simulink model "IEEE13bus_1subsystem"  (R2022b)
settings: Solver=ode4  StartTime=0.0  StopTime=inf  FixedStep=Ts  MaxStep=1e-4  RelTol=1e-4
InitFcn:
  | a=1; % Loading Factor
  | Ts=50e-6;
  | % phase to sequence conversion of RXB matrices
  | c=1*exp(sqrt(-1)*(120*pi/180));
  | T=[1 1 1;1 c*c c;1 c c*c];
  | Tinv=1/3*[1 1 1;1 c c*c;1 c*c c];
  | 
  | % Simulation data for the IEEE 13 Node Test Feeder model
  | mi2km = 1.60934;%  miles to km conversion
  | ft2km = 0.0003048; % feet to km conversion
  | ms2F = 1*1e-6/(2*pi*60);% microsiemens to Farads conversion
  | 
  | 
  | %% Configuration 601
  | % Series Resitance and Reactance - ohm/mile
  | R_601 = [0.3465 0.1560 0.1580;0.1560 0.3375 0.1535;0.1580 0.1535 0.3414];
  | X_601 = [1.1079 0.5017 0.4236;0.5017 1.0478 0.3849;0.4236 0.3849 1.0348];
  | % charging susceptance - microsiemens/mile
  | B_601 = [6.2998 -1.9958 -1.2595;-1.9958 5.9597 -0.7417;-1.2595 -0.7417 5.6386];
  | 
  | R_601 = R_601/mi2km;
  | Rseq=Tinv*R_601*T;
  | R1_601=Rseq(2,2);R0_601=Rseq(1,1);
  | 
  | L_601 = (X_601/(2*pi*60))/mi2km;
  | Lseq=Tinv*L_601*T;
  | L1_601=Lseq(2,2);L0_601=Lseq(1,1);
  | 
  | C_601 =(B_601*ms2F)/mi2km;
  | Cseq=Tinv*C_601*T;
  | C1_601=Cseq(2,2);C0_601=Cseq(1,1);
  | 
  | %% Configuration 602 - series reactance - ohm/mile
  | R_602 = [0.7526 0.1580 0.1560;0.1580 0.7475 0.1535;0.1560 0.1535 0.7436];
  | X_602 = [1.1814 0.4236 0.5017;0.4236 1.1983 0.3849;0.5017 0.3849 1.2112];
  | % charging susceptance - microsiemens/mile
  | B_602 = [5.6990 -1.0817 -1.6905;-1.0817 5.1795 -0.6588;-1.6905 -0.6588 5.4246];
  | 
  | R_602 = R_602/mi2km;
  | Rseq=Tinv*R_602*T;
  | R1_602=Rseq(2,2);R0_602=Rseq(1,1);
  | 
  | L_602 = (X_602/(2*pi*60))/mi2km;
  | Lseq=Tinv*L_602*T;
  | L1_602=Lseq(2,2);L0_602=Lseq(1,1);
  | 
  | C_602 =(B_602*ms2F)/mi2km;
  | Cseq=Tinv*C_602*T;
  | C1_602=Cseq(2,2);C0_602=Cseq(1,1);
  | %% Configuration 603 - series reactance - ohm/mile
  | R_603 = [0 0 0;0 1.3294 0.2066;0 0.2066 1.3238];
  | X_603 = [0 0 0;0 1.3471 0.4591;0 0.4591 1.3569];
  | % charging susceptance - microsiemens/mile
  | B_603 = [0 0 0;0 4.7097 -0.8999;0 -0.8999 4.6658];
  | 
  | % convert for SPS
  | R_603 = R_603/mi2km;
  | Rseq=Tinv*R_603*T;
  | R1_603=Rseq(2,2);R0_603=Rseq(1,1);
  | 
  | ... (+71 lines)
undefined symbols (not defined in the file): find_system, I, Left, MOV_segment9, powergui, Right, type, V, X
libraries: spsSeriesRLCBranchLib x57, spsGroundLib x42, spsVoltageMeasurementLib x18, spsThreePhaseVIMeasurementLib x16, spsDCVoltageSourceLib x12, spsThreePhaseSeriesRLCLoadLib x7, ssn_lib x6, spsACCurrentSourceLib x6, spsOnDelayLib x6, spsThreePhasePISectionLineLib x5, spsSeriesRLCLoadLib x5, spsRMSLib x4
(part 4 of 4)

== system IEEE13bus_1subsystem/SM_13p/Regulator 1/Single Phase SVR_A2/Voltage Regulator Control/Tap Changer Control ==
  "Up " : Inport
  "Down " : Inport  Port=2
  Constant : Constant  Value=-1
  Constant1 : Constant
  Determine tap position : Subsystem
  Edge Detector : Subsystem  DialogController=POWERSYS.PowerSysDialog  mask(Edge Detector){model=Rising, ic=0}
      mask prompts: model "Edge:"; ic "Input at t = -eps:"
      mask help:
      | This block compares its present input to its previous input.
      |
      | If the input  is a logic signal (TRUE (1) or FALSE (0), the output is a one-step boolean signal TRUE  when  the specified edge (Rising, Falling or Either)  is detected.
      |
      | This block can also be used to detect the slope polarity of a continuous signal. For example, if the specified edge is  "Rising", the output is TRUE as long as the slope of the input signal is positive.
      |
      | The input value at time preceding t=0 is specified by the parameter "Input at t=-eps"
      mask init: same as IEEE13bus_1subsystem/SM_13p/Regulator 1/Single Phase SVR_A/Voltage Regulator Control/Tap Changer Control/Edge Detector
      mask Help: This block is part of a subset of blocks in the Extras library that does not have documentation associated with it, other than the block mask description.
      mask TypeOptions model: Rising | Falling | Either
      mask Display: plot(0,0,100,100, X1,Y1,X2,Y2,X3,Y3,X4,Y4);
  Logical Operator : Logic  Operator=OR  AllPortsSameDT=off
  Logical Operator1 : Logic  AllPortsSameDT=off
  Mechanical Delay : TransportDelay  DelayTime=MecDelay  InitialOutput=InitialPosition  BufferSize=5120
  Memory : Memory  InitialCondition=1  InheritSampleTime=on
  Relational Operator : RelationalOperator  Operator===  OutDataTypeStr=float('double')  InputSameDT=off
  Switch : Switch  Threshold=0.5  InputSameDT=off
  TapNo : Outport  VectorParamsAs1DForOutWhenUnconnected=off
  Ready : Outport  Port=2  VectorParamsAs1DForOutWhenUnconnected=off
  wires:
  Mechanical Delay/1 -> TapNo/1, Relational Operator/2
  Logical Operator1/1 -> Determine tap position/Trigger
  "Up "/1 -> Logical Operator/1
  "Down "/1 -> Logical Operator/2, Switch/2
  Constant/1 -> Switch/1
  Constant1/1 -> Switch/3
  Switch/1 -> Determine tap position/1(NewTap)
  Determine tap position/1(TapNo) -> Mechanical Delay/1, Relational Operator/1
  Relational Operator/1 -> Memory/1
  Memory/1 -> Logical Operator1/1, Ready/1
  Logical Operator/1 -> Edge Detector/1(In)
  Edge Detector/1(Out) -> Logical Operator1/2

== system IEEE13bus_1subsystem/SM_13p/Regulator 1/Single Phase SVR_A2/Voltage Regulator Control/Voltage regulator ==
  Vmes (pu) : Inport
  Ready : Inport  Port=2
  RegOn : Inport  Port=3
  Dead Zone : DeadZone  LowerValue=-DeadBand/2  UpperValue=+DeadBand/2
  Discrete Variable Time Delay : spsDiscreteVariableTimeDelayLib/Discrete Variable Time Delay  MaxDelay=3/60+Ts  InitialValue=1  Ts=Ts  DFT=on
      settings: LibrarySourceBlock=|
      | sps_lib/Control/Discrete Variable
      | Time Delay
  Logical Operator : Logic  AllPortsSameDT=off
  Logical Operator1 : Logic  AllPortsSameDT=off
  On Delay : spsOnDelayLib/On Delay  DelayType=On delay  delay=TimeDelay  ic=0  Ts=Ts
  On Delay1 : spsOnDelayLib/On Delay  DelayType=On delay  delay=TimeDelay  ic=0  Ts=Ts
  Relational Operator : RelationalOperator  Operator=>  InputSameDT=off
  Relational Operator1 : RelationalOperator  Operator=<  InputSameDT=off
  Sum : Sum  Inputs=|+-  SaturateOnIntegerOverflow=on
  Switch : Switch  Threshold=1.5  InputSameDT=off
  Vref : Constant  Value=Vref
  Vref1 : Constant  Value=0
  Vref2 : Constant  Value=0
  Vref3 : Constant  Value=0
  Vref4 : Constant  Value=3/60
  Up : Outport  VectorParamsAs1DForOutWhenUnconnected=off
  Down : Outport  Port=2  VectorParamsAs1DForOutWhenUnconnected=off
  wires:
  Vref2/1 -> Switch/3
  RegOn/1 -> Switch/2
  Switch/1 -> Dead Zone/1
  Sum/1 -> Switch/1
  Vref/1 -> Sum/1
  Vmes (pu)/1 -> Sum/2
  Dead Zone/1 -> Relational Operator1/1, Relational Operator/1
  Vref1/1 -> Relational Operator/2
  Relational Operator/1 -> Logical Operator/1
  Ready/1 -> Discrete Variable Time Delay/1
  Logical Operator/1 -> On Delay/1
  On Delay/1 -> Up/1
  Relational Operator1/1 -> Logical Operator1/2
  Logical Operator1/1 -> On Delay1/1
  On Delay1/1 -> Down/1
  Vref3/1 -> Relational Operator1/2
  Discrete Variable Time Delay/1 -> Logical Operator1/1, Logical Operator/2
  Vref4/1 -> Discrete Variable Time Delay/2

== system IEEE13bus_1subsystem/SM_13p/Regulator 1/Single Phase SVR_A/Transformer with Taps/SSN OLTC xfo v2/DC source_a ==
  I1A_V : spsDCVoltageSourceLib/DC Voltage Source  Amplitude=0  Measurements=None
  Conn1 : PMIOPort  Side=Left
  Conn2 : PMIOPort  Port=2  Side=Right
  connections:
  Conn2/RConn1 -- I1A_V/RConn1
  Conn1/RConn1 -- I1A_V/LConn1

== system IEEE13bus_1subsystem/SM_13p/Regulator 1/Single Phase SVR_A/Transformer with Taps/SSN OLTC xfo v2/DC source_b ==
  I1B_V : spsDCVoltageSourceLib/DC Voltage Source  Amplitude=0  Measurements=None
  Conn3 : PMIOPort  Side=Left
  Conn4 : PMIOPort  Port=2  Side=Right
  connections:
  Conn3/RConn1 -- I1B_V/LConn1
  Conn4/RConn1 -- I1B_V/RConn1

== system IEEE13bus_1subsystem/SM_13p/Regulator 1/Single Phase SVR_A/Transformer with Taps/SSN OLTC xfo v2/DC source_c ==
  I1C_V : spsDCVoltageSourceLib/DC Voltage Source  Amplitude=0  Measurements=None
  Conn1 : PMIOPort  Side=Left
  Conn2 : PMIOPort  Port=2  Side=Right
  connections:
  Conn1/RConn1 -- I1C_V/LConn1
  Conn2/RConn1 -- I1C_V/RConn1

== system IEEE13bus_1subsystem/SM_13p/Regulator 1/Single Phase SVR_A/Transformer with Taps/SSN OLTC xfo v2/DC source_d ==
  I1D_V : spsDCVoltageSourceLib/DC Voltage Source  Amplitude=0  Measurements=None
  Conn3 : PMIOPort  Side=Left
  Conn4 : PMIOPort  Port=2  Side=Right
  connections:
  Conn4/RConn1 -- I1D_V/RConn1
  Conn3/RConn1 -- I1D_V/LConn1

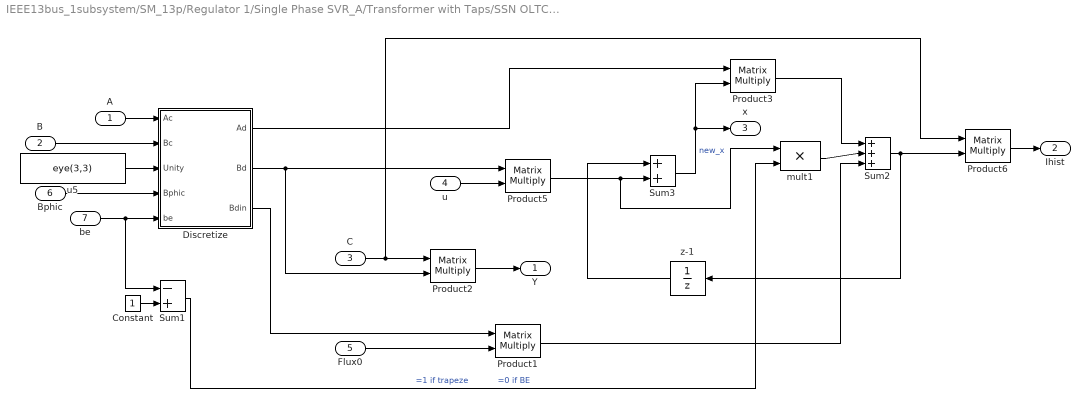
== system IEEE13bus_1subsystem/SM_13p/Regulator 1/Single Phase SVR_A/Transformer with Taps/SSN OLTC xfo v2/SSS-SM equations ==
  A : Inport
  B : Inport  Port=2
  C : Inport  Port=3
  u : Inport  Port=4
  Flux0 : Inport  Port=5
  Bphic : Inport  Port=6
  be : Inport  Port=7
  Constant : Constant
  Discretize : Subsystem
  Product{1..3,5..6} (5 alike) : Product  Multiplication=Matrix(*)  SaturateOnIntegerOverflow=on  OutDataTypeStr=Inherit: Same as first input
  Sum1 : Sum  Inputs=-+  SaturateOnIntegerOverflow=on
  Sum2 : Sum  Inputs=+++  SaturateOnIntegerOverflow=on
  Sum3 : Sum  SaturateOnIntegerOverflow=on
  mult1 : Product
  u5 : Constant  Value=eye(3,3)
  z-1 : UnitDelay  SampleTime=Ts  HasFrameUpgradeWarning=on
  Y : Outport  VectorParamsAs1DForOutWhenUnconnected=off
  Ihist : Outport  Port=2  VectorParamsAs1DForOutWhenUnconnected=off
  x : Outport  Port=3  VectorParamsAs1DForOutWhenUnconnected=off
  wires:
  be/1 -> Sum1/1, Discretize/5(be)
  Sum1/1 -> mult1/2  "=1 if trapeze           =0 if BE"
  mult1/1 -> Sum2/2
  Constant/1 -> Sum1/2
  Bphic/1 -> Discretize/4(Bphic)
  Flux0/1 -> Product1/2
  Product1/1 -> Sum2/3
  Discretize/3(Bdin) -> Product1/1
  Discretize/2(Bd) -> Product2/2, Product5/1
  z-1/1 -> Sum3/1
  u/1 -> Product5/2
  Discretize/1(Ad) -> Product3/1
  Sum2/1 -> Product6/2, z-1/1
  Sum3/1 -> x/1, Product3/2  "new_x"
  Product3/1 -> Sum2/1
  Product5/1 -> mult1/1, Sum3/2
  Product6/1 -> Ihist/1
  C/1 -> Product6/1, Product2/1
  B/1 -> Discretize/2(Bc)
  A/1 -> Discretize/1(Ac)
  Product2/1 -> Y/1
  u5/1 -> Discretize/3(Unity)

== system IEEE13bus_1subsystem/SM_13p/Regulator 1/Single Phase SVR_A/Transformer with Taps/SSN OLTC xfo v2/Update Matrix L ==
  k : Inport
  L2 : Inport  Port=2
  Lin : Inport  Port=3
  "L2->(2,2) " : Assignment  NumberOfDimensions=2  IndexOptions=Index vector (dialog),Index vector (dialog)  Indices=[2],[2]  OutputSizes=1,1
  k->(2,3) : Assignment  NumberOfDimensions=2  IndexOptions=Index vector (dialog),Index vector (dialog)  Indices=[2],[3]  OutputSizes=1,1
  L : Outport  VectorParamsAs1DForOutWhenUnconnected=off
  wires:
  k->(2,3)/1 -> "L2->(2,2) "/1
  k/1 -> k->(2,3)/2
  Lin/1 -> k->(2,3)/1
  L2/1 -> "L2->(2,2) "/2
  "L2->(2,2) "/1 -> L/1

== system IEEE13bus_1subsystem/SM_13p/Regulator 1/Single Phase SVR_A/Transformer with Taps/SSN OLTC xfo v2/Update Matrix R ==
  R2 : Inport
  Rin : Inport  Port=2
  k : Inport  Port=3
  Rcore : Inport  Port=4
  Rcore/Lcore : Inport  Port=5
  "-R2->(2,2) " : Assignment  NumberOfDimensions=2  IndexOptions=Index vector (dialog),Index vector (dialog)  Indices=[2],[2]  OutputSizes=1,1
  -Rm/Lm->(3,3) : Assignment  NumberOfDimensions=2  IndexOptions=Index vector (dialog),Index vector (dialog)  Indices=3,3  OutputSizes=1,1
  Gain : Gain  Gain=-1
  Gain1 : Gain  Gain=-1
  Product1 : Product  RndMeth=Zero
  kRm->(3,2) : Assignment  NumberOfDimensions=2  IndexOptions=Index vector (dialog),Index vector (dialog)  Indices=3,2  OutputSizes=1,1
  R : Outport  VectorParamsAs1DForOutWhenUnconnected=off
  wires:
  Rcore/Lcore/1 -> Gain1/1
  Gain1/1 -> -Rm/Lm->(3,3)/2
  Rcore/1 -> Product1/1
  -Rm/Lm->(3,3)/1 -> R/1
  kRm->(3,2)/1 -> -Rm/Lm->(3,3)/1
  Product1/1 -> kRm->(3,2)/2
  k/1 -> Product1/2
  Gain/1 -> "-R2->(2,2) "/2
  Rin/1 -> "-R2->(2,2) "/1
  R2/1 -> Gain/1
  "-R2->(2,2) "/1 -> kRm->(3,2)/1

== system IEEE13bus_1subsystem/SM_13p/Regulator 1/Single Phase SVR_A/Transformer with Taps/SSN OLTC xfo v2/conn_down_c ==
  b2 : PMIOPort  Side=Right
  b1 : PMIOPort  Port=2  Side=Left
  connections:
  b1/RConn1 -- b2/RConn1

== system IEEE13bus_1subsystem/SM_13p/Regulator 1/Single Phase SVR_A/Transformer with Taps/SSN OLTC xfo v2/conn_down_d ==
  b2 : PMIOPort  Side=Right
  b1 : PMIOPort  Port=2  Side=Left
  connections:
  b1/RConn1 -- b2/RConn1

== system IEEE13bus_1subsystem/SM_13p/Regulator 1/Single Phase SVR_A/Transformer with Taps/SSN OLTC xfo v2/conn_up_c ==
  b2 : PMIOPort  Side=Right
  b1 : PMIOPort  Port=2  Side=Left
  connections:
  b1/RConn1 -- b2/RConn1

== system IEEE13bus_1subsystem/SM_13p/Regulator 1/Single Phase SVR_A/Transformer with Taps/SSN OLTC xfo v2/conn_up_d ==
  b2 : PMIOPort  Side=Right
  b1 : PMIOPort  Port=2  Side=Left
  connections:
  b1/RConn1 -- b2/RConn1

== system IEEE13bus_1subsystem/SM_13p/Regulator 1/Single Phase SVR_A/Voltage Regulator Control/Tap Changer Control/Determine tap position ==
  NewTap : Inport
  Trigger : TriggerPort  VariantControl=Variant
  Memory : Memory  InitialCondition=InitialPosition  InheritSampleTime=on
  Saturation : Saturate  UpperLimit=MinMaxTap(2)  LowerLimit=MinMaxTap(1)
  Sum : Sum  Inputs=|++  SaturateOnIntegerOverflow=on
  TapNo : Outport  InitialOutput=InitialPosition  VectorParamsAs1DForOutWhenUnconnected=off
  wires:
  NewTap/1 -> Sum/1
  Sum/1 -> Saturation/1
  Memory/1 -> Sum/2
  Saturation/1 -> TapNo/1, Memory/1

== system IEEE13bus_1subsystem/SM_13p/Regulator 1/Single Phase SVR_A/Voltage Regulator Control/Tap Changer Control/Edge Detector ==
  note: Edge or Slope Detector
  In : Inport
  Constant1 : Constant  Value=model
  Demux : Demux  Outputs=2
      settings: DisplayOption=none
  Logical Operator1 : Logic  Operator=OR
  Memory : Memory  InitialCondition=ic  LinearizeAsDelay=on
  Multiport Switch : MultiPortSwitch  InputSameDT=off
  NEGATIVE Edge : Subsystem  TreatAsAtomicUnit=on
  POSITIVE Edge : Subsystem  TreatAsAtomicUnit=on
  either edge : Constant  Value=[1 1]
  neg. edge : Constant  Value=[0 1]
  pos. edge : Constant  Value=[1 0]
  Out : Outport  VectorParamsAs1DForOutWhenUnconnected=off
  wires:
  either edge/1 -> Multiport Switch/4
  Demux/2 -> NEGATIVE Edge/Enable
  Demux/1 -> POSITIVE Edge/Enable
  Multiport Switch/1 -> Demux/1
  Constant1/1 -> Multiport Switch/1
  neg. edge/1 -> Multiport Switch/3
  pos. edge/1 -> Multiport Switch/2
  In/1 -> Memory/1, NEGATIVE Edge/1(IN), POSITIVE Edge/1(IN)
  Memory/1 -> NEGATIVE Edge/2(IN previous), POSITIVE Edge/2(IN previous)
  POSITIVE Edge/1(OUT) -> Logical Operator1/1
  NEGATIVE Edge/1(OUT) -> Logical Operator1/2
  Logical Operator1/1 -> Out/1

== system IEEE13bus_1subsystem/SM_13p/Regulator 1/Single Phase SVR_A1/Transformer with Taps/SSN OLTC xfo v2/DC source_a ==
  I1A_V : spsDCVoltageSourceLib/DC Voltage Source  Amplitude=0  Measurements=None
  Conn1 : PMIOPort  Side=Left
  Conn2 : PMIOPort  Port=2  Side=Right
  connections:
  Conn1/RConn1 -- I1A_V/LConn1
  Conn2/RConn1 -- I1A_V/RConn1

== system IEEE13bus_1subsystem/SM_13p/Regulator 1/Single Phase SVR_A1/Transformer with Taps/SSN OLTC xfo v2/DC source_b ==
  I1B_V : spsDCVoltageSourceLib/DC Voltage Source  Amplitude=0  Measurements=None
  Conn3 : PMIOPort  Side=Left
  Conn4 : PMIOPort  Port=2  Side=Right
  connections:
  Conn4/RConn1 -- I1B_V/RConn1
  Conn3/RConn1 -- I1B_V/LConn1

== system IEEE13bus_1subsystem/SM_13p/Regulator 1/Single Phase SVR_A1/Transformer with Taps/SSN OLTC xfo v2/DC source_c ==
  I1C_V : spsDCVoltageSourceLib/DC Voltage Source  Amplitude=0  Measurements=None
  Conn1 : PMIOPort  Side=Left
  Conn2 : PMIOPort  Port=2  Side=Right
  connections:
  Conn2/RConn1 -- I1C_V/RConn1
  Conn1/RConn1 -- I1C_V/LConn1

== system IEEE13bus_1subsystem/SM_13p/Regulator 1/Single Phase SVR_A1/Transformer with Taps/SSN OLTC xfo v2/DC source_d ==
  I1D_V : spsDCVoltageSourceLib/DC Voltage Source  Amplitude=0  Measurements=None
  Conn3 : PMIOPort  Side=Left
  Conn4 : PMIOPort  Port=2  Side=Right
  connections:
  Conn3/RConn1 -- I1D_V/LConn1
  Conn4/RConn1 -- I1D_V/RConn1

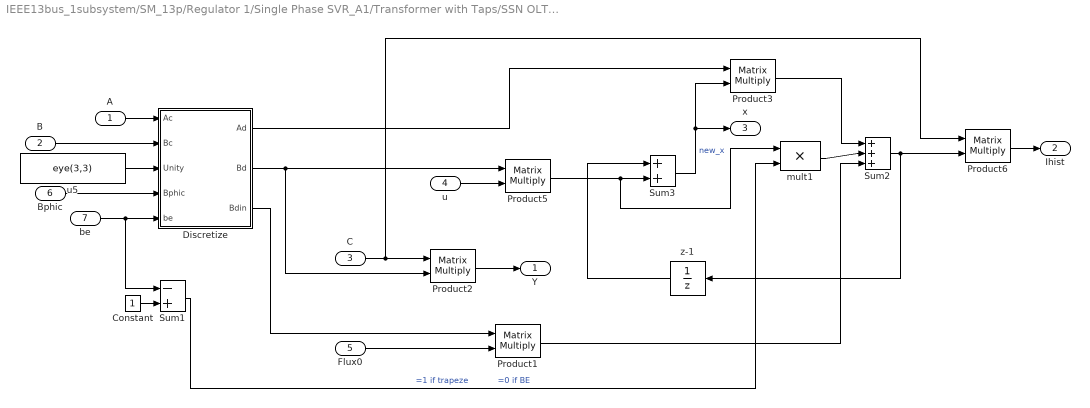
== system IEEE13bus_1subsystem/SM_13p/Regulator 1/Single Phase SVR_A1/Transformer with Taps/SSN OLTC xfo v2/SSS-SM equations ==
  A : Inport
  B : Inport  Port=2
  C : Inport  Port=3
  u : Inport  Port=4
  Flux0 : Inport  Port=5
  Bphic : Inport  Port=6
  be : Inport  Port=7
  Constant : Constant
  Discretize : Subsystem
  Product{1..3,5..6} (5 alike) : Product  Multiplication=Matrix(*)  SaturateOnIntegerOverflow=on  OutDataTypeStr=Inherit: Same as first input
  Sum1 : Sum  Inputs=-+  SaturateOnIntegerOverflow=on
  Sum2 : Sum  Inputs=+++  SaturateOnIntegerOverflow=on
  Sum3 : Sum  SaturateOnIntegerOverflow=on
  mult1 : Product
  u5 : Constant  Value=eye(3,3)
  z-1 : UnitDelay  SampleTime=Ts  HasFrameUpgradeWarning=on
  Y : Outport  VectorParamsAs1DForOutWhenUnconnected=off
  Ihist : Outport  Port=2  VectorParamsAs1DForOutWhenUnconnected=off
  x : Outport  Port=3  VectorParamsAs1DForOutWhenUnconnected=off
  wires:
  u5/1 -> Discretize/3(Unity)
  Product2/1 -> Y/1
  A/1 -> Discretize/1(Ac)
  B/1 -> Discretize/2(Bc)
  C/1 -> Product2/1, Product6/1
  Product6/1 -> Ihist/1
  Product5/1 -> Sum3/2, mult1/1
  Product3/1 -> Sum2/1
  Sum3/1 -> Product3/2, x/1  "new_x"
  Sum2/1 -> z-1/1, Product6/2
  Discretize/1(Ad) -> Product3/1
  u/1 -> Product5/2
  z-1/1 -> Sum3/1
  Discretize/2(Bd) -> Product5/1, Product2/2
  Discretize/3(Bdin) -> Product1/1
  Product1/1 -> Sum2/3
  Flux0/1 -> Product1/2
  Bphic/1 -> Discretize/4(Bphic)
  Constant/1 -> Sum1/2
  mult1/1 -> Sum2/2
  Sum1/1 -> mult1/2  "=1 if trapeze           =0 if BE"
  be/1 -> Discretize/5(be), Sum1/1

== system IEEE13bus_1subsystem/SM_13p/Regulator 1/Single Phase SVR_A1/Transformer with Taps/SSN OLTC xfo v2/Update Matrix L ==
  k : Inport
  L2 : Inport  Port=2
  Lin : Inport  Port=3
  "L2->(2,2) " : Assignment  NumberOfDimensions=2  IndexOptions=Index vector (dialog),Index vector (dialog)  Indices=[2],[2]  OutputSizes=1,1
  k->(2,3) : Assignment  NumberOfDimensions=2  IndexOptions=Index vector (dialog),Index vector (dialog)  Indices=[2],[3]  OutputSizes=1,1
  L : Outport  VectorParamsAs1DForOutWhenUnconnected=off
  wires:
  "L2->(2,2) "/1 -> L/1
  L2/1 -> "L2->(2,2) "/2
  Lin/1 -> k->(2,3)/1
  k/1 -> k->(2,3)/2
  k->(2,3)/1 -> "L2->(2,2) "/1

== system IEEE13bus_1subsystem/SM_13p/Regulator 1/Single Phase SVR_A1/Transformer with Taps/SSN OLTC xfo v2/Update Matrix R ==
  R2 : Inport
  Rin : Inport  Port=2
  k : Inport  Port=3
  Rcore : Inport  Port=4
  Rcore/Lcore : Inport  Port=5
  "-R2->(2,2) " : Assignment  NumberOfDimensions=2  IndexOptions=Index vector (dialog),Index vector (dialog)  Indices=[2],[2]  OutputSizes=1,1
  -Rm/Lm->(3,3) : Assignment  NumberOfDimensions=2  IndexOptions=Index vector (dialog),Index vector (dialog)  Indices=3,3  OutputSizes=1,1
  Gain : Gain  Gain=-1
  Gain1 : Gain  Gain=-1
  Product1 : Product  RndMeth=Zero
  kRm->(3,2) : Assignment  NumberOfDimensions=2  IndexOptions=Index vector (dialog),Index vector (dialog)  Indices=3,2  OutputSizes=1,1
  R : Outport  VectorParamsAs1DForOutWhenUnconnected=off
  wires:
  "-R2->(2,2) "/1 -> kRm->(3,2)/1
  R2/1 -> Gain/1
  Rin/1 -> "-R2->(2,2) "/1
  Gain/1 -> "-R2->(2,2) "/2
  k/1 -> Product1/2
  Product1/1 -> kRm->(3,2)/2
  kRm->(3,2)/1 -> -Rm/Lm->(3,3)/1
  -Rm/Lm->(3,3)/1 -> R/1
  Rcore/1 -> Product1/1
  Gain1/1 -> -Rm/Lm->(3,3)/2
  Rcore/Lcore/1 -> Gain1/1

== system IEEE13bus_1subsystem/SM_13p/Regulator 1/Single Phase SVR_A1/Transformer with Taps/SSN OLTC xfo v2/conn_down_c ==
  b2 : PMIOPort  Side=Right
  b1 : PMIOPort  Port=2  Side=Left
  connections:
  b1/RConn1 -- b2/RConn1

== system IEEE13bus_1subsystem/SM_13p/Regulator 1/Single Phase SVR_A1/Transformer with Taps/SSN OLTC xfo v2/conn_down_d ==
  b2 : PMIOPort  Side=Right
  b1 : PMIOPort  Port=2  Side=Left
  connections:
  b1/RConn1 -- b2/RConn1

== system IEEE13bus_1subsystem/SM_13p/Regulator 1/Single Phase SVR_A1/Transformer with Taps/SSN OLTC xfo v2/conn_up_c ==
  b2 : PMIOPort  Side=Right
  b1 : PMIOPort  Port=2  Side=Left
  connections:
  b1/RConn1 -- b2/RConn1

== system IEEE13bus_1subsystem/SM_13p/Regulator 1/Single Phase SVR_A1/Transformer with Taps/SSN OLTC xfo v2/conn_up_d ==
  b2 : PMIOPort  Side=Right
  b1 : PMIOPort  Port=2  Side=Left
  connections:
  b1/RConn1 -- b2/RConn1

== system IEEE13bus_1subsystem/SM_13p/Regulator 1/Single Phase SVR_A1/Voltage Regulator Control/Tap Changer Control/Determine tap position ==
  NewTap : Inport
  Trigger : TriggerPort  VariantControl=Variant
  Memory : Memory  InitialCondition=InitialPosition  InheritSampleTime=on
  Saturation : Saturate  UpperLimit=MinMaxTap(2)  LowerLimit=MinMaxTap(1)
  Sum : Sum  Inputs=|++  SaturateOnIntegerOverflow=on
  TapNo : Outport  InitialOutput=InitialPosition  VectorParamsAs1DForOutWhenUnconnected=off
  wires:
  Saturation/1 -> Memory/1, TapNo/1
  Memory/1 -> Sum/2
  Sum/1 -> Saturation/1
  NewTap/1 -> Sum/1

== system IEEE13bus_1subsystem/SM_13p/Regulator 1/Single Phase SVR_A1/Voltage Regulator Control/Tap Changer Control/Edge Detector ==
  note: Edge or Slope Detector
  In : Inport
  Constant1 : Constant  Value=model
  Demux : Demux  Outputs=2
      settings: DisplayOption=none
  Logical Operator1 : Logic  Operator=OR
  Memory : Memory  InitialCondition=ic  LinearizeAsDelay=on
  Multiport Switch : MultiPortSwitch  InputSameDT=off
  NEGATIVE Edge : Subsystem  TreatAsAtomicUnit=on
  POSITIVE Edge : Subsystem  TreatAsAtomicUnit=on
  either edge : Constant  Value=[1 1]
  neg. edge : Constant  Value=[0 1]
  pos. edge : Constant  Value=[1 0]
  Out : Outport  VectorParamsAs1DForOutWhenUnconnected=off
  wires:
  Logical Operator1/1 -> Out/1
  NEGATIVE Edge/1(OUT) -> Logical Operator1/2
  POSITIVE Edge/1(OUT) -> Logical Operator1/1
  Memory/1 -> POSITIVE Edge/2(IN previous), NEGATIVE Edge/2(IN previous)
  In/1 -> POSITIVE Edge/1(IN), NEGATIVE Edge/1(IN), Memory/1
  pos. edge/1 -> Multiport Switch/2
  neg. edge/1 -> Multiport Switch/3
  Constant1/1 -> Multiport Switch/1
  Multiport Switch/1 -> Demux/1
  Demux/1 -> POSITIVE Edge/Enable
  Demux/2 -> NEGATIVE Edge/Enable
  either edge/1 -> Multiport Switch/4

== system IEEE13bus_1subsystem/SM_13p/Regulator 1/Single Phase SVR_A2/Transformer with Taps/SSN OLTC xfo v2/DC source_a ==
  I1A_V : spsDCVoltageSourceLib/DC Voltage Source  Amplitude=0  Measurements=None
  Conn1 : PMIOPort  Side=Left
  Conn2 : PMIOPort  Port=2  Side=Right
  connections:
  Conn2/RConn1 -- I1A_V/RConn1
  Conn1/RConn1 -- I1A_V/LConn1

== system IEEE13bus_1subsystem/SM_13p/Regulator 1/Single Phase SVR_A2/Transformer with Taps/SSN OLTC xfo v2/DC source_b ==
  I1B_V : spsDCVoltageSourceLib/DC Voltage Source  Amplitude=0  Measurements=None
  Conn3 : PMIOPort  Side=Left
  Conn4 : PMIOPort  Port=2  Side=Right
  connections:
  Conn3/RConn1 -- I1B_V/LConn1
  Conn4/RConn1 -- I1B_V/RConn1

== system IEEE13bus_1subsystem/SM_13p/Regulator 1/Single Phase SVR_A2/Transformer with Taps/SSN OLTC xfo v2/DC source_c ==
  I1C_V : spsDCVoltageSourceLib/DC Voltage Source  Amplitude=0  Measurements=None
  Conn1 : PMIOPort  Side=Left
  Conn2 : PMIOPort  Port=2  Side=Right
  connections:
  Conn1/RConn1 -- I1C_V/LConn1
  Conn2/RConn1 -- I1C_V/RConn1

== system IEEE13bus_1subsystem/SM_13p/Regulator 1/Single Phase SVR_A2/Transformer with Taps/SSN OLTC xfo v2/DC source_d ==
  I1D_V : spsDCVoltageSourceLib/DC Voltage Source  Amplitude=0  Measurements=None
  Conn3 : PMIOPort  Side=Left
  Conn4 : PMIOPort  Port=2  Side=Right
  connections:
  Conn4/RConn1 -- I1D_V/RConn1
  Conn3/RConn1 -- I1D_V/LConn1

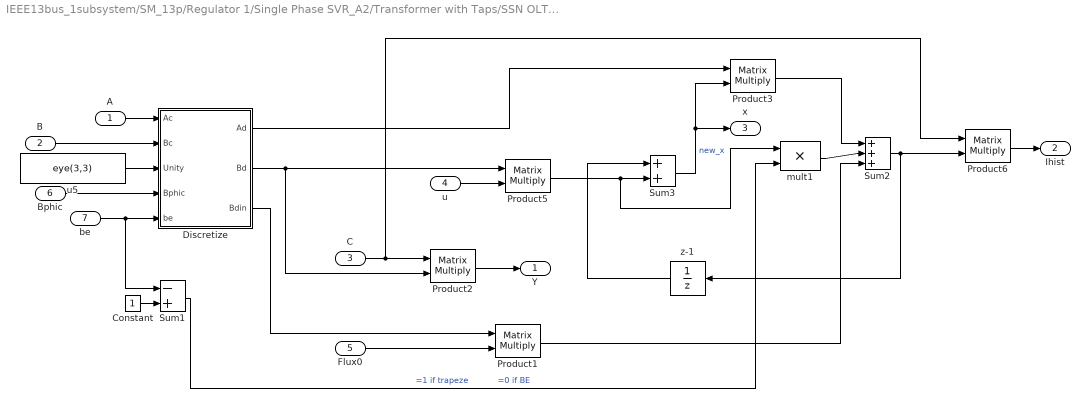
== system IEEE13bus_1subsystem/SM_13p/Regulator 1/Single Phase SVR_A2/Transformer with Taps/SSN OLTC xfo v2/SSS-SM equations ==
  A : Inport
  B : Inport  Port=2
  C : Inport  Port=3
  u : Inport  Port=4
  Flux0 : Inport  Port=5
  Bphic : Inport  Port=6
  be : Inport  Port=7
  Constant : Constant
  Discretize : Subsystem
  Product{1..3,5..6} (5 alike) : Product  Multiplication=Matrix(*)  SaturateOnIntegerOverflow=on  OutDataTypeStr=Inherit: Same as first input
  Sum1 : Sum  Inputs=-+  SaturateOnIntegerOverflow=on
  Sum2 : Sum  Inputs=+++  SaturateOnIntegerOverflow=on
  Sum3 : Sum  SaturateOnIntegerOverflow=on
  mult1 : Product
  u5 : Constant  Value=eye(3,3)
  z-1 : UnitDelay  SampleTime=Ts  HasFrameUpgradeWarning=on
  Y : Outport  VectorParamsAs1DForOutWhenUnconnected=off
  Ihist : Outport  Port=2  VectorParamsAs1DForOutWhenUnconnected=off
  x : Outport  Port=3  VectorParamsAs1DForOutWhenUnconnected=off
  wires:
  be/1 -> Sum1/1, Discretize/5(be)
  Sum1/1 -> mult1/2  "=1 if trapeze           =0 if BE"
  mult1/1 -> Sum2/2
  Constant/1 -> Sum1/2
  Bphic/1 -> Discretize/4(Bphic)
  Flux0/1 -> Product1/2
  Product1/1 -> Sum2/3
  Discretize/3(Bdin) -> Product1/1
  Discretize/2(Bd) -> Product2/2, Product5/1
  z-1/1 -> Sum3/1
  u/1 -> Product5/2
  Discretize/1(Ad) -> Product3/1
  Sum2/1 -> Product6/2, z-1/1
  Sum3/1 -> x/1, Product3/2  "new_x"
  Product3/1 -> Sum2/1
  Product5/1 -> mult1/1, Sum3/2
  Product6/1 -> Ihist/1
  C/1 -> Product6/1, Product2/1
  B/1 -> Discretize/2(Bc)
  A/1 -> Discretize/1(Ac)
  Product2/1 -> Y/1
  u5/1 -> Discretize/3(Unity)

== system IEEE13bus_1subsystem/SM_13p/Regulator 1/Single Phase SVR_A2/Transformer with Taps/SSN OLTC xfo v2/Update Matrix L ==
  k : Inport
  L2 : Inport  Port=2
  Lin : Inport  Port=3
  "L2->(2,2) " : Assignment  NumberOfDimensions=2  IndexOptions=Index vector (dialog),Index vector (dialog)  Indices=[2],[2]  OutputSizes=1,1
  k->(2,3) : Assignment  NumberOfDimensions=2  IndexOptions=Index vector (dialog),Index vector (dialog)  Indices=[2],[3]  OutputSizes=1,1
  L : Outport  VectorParamsAs1DForOutWhenUnconnected=off
  wires:
  k->(2,3)/1 -> "L2->(2,2) "/1
  k/1 -> k->(2,3)/2
  Lin/1 -> k->(2,3)/1
  L2/1 -> "L2->(2,2) "/2
  "L2->(2,2) "/1 -> L/1

== system IEEE13bus_1subsystem/SM_13p/Regulator 1/Single Phase SVR_A2/Transformer with Taps/SSN OLTC xfo v2/Update Matrix R ==
  R2 : Inport
  Rin : Inport  Port=2
  k : Inport  Port=3
  Rcore : Inport  Port=4
  Rcore/Lcore : Inport  Port=5
  "-R2->(2,2) " : Assignment  NumberOfDimensions=2  IndexOptions=Index vector (dialog),Index vector (dialog)  Indices=[2],[2]  OutputSizes=1,1
  -Rm/Lm->(3,3) : Assignment  NumberOfDimensions=2  IndexOptions=Index vector (dialog),Index vector (dialog)  Indices=3,3  OutputSizes=1,1
  Gain : Gain  Gain=-1
  Gain1 : Gain  Gain=-1
  Product1 : Product  RndMeth=Zero
  kRm->(3,2) : Assignment  NumberOfDimensions=2  IndexOptions=Index vector (dialog),Index vector (dialog)  Indices=3,2  OutputSizes=1,1
  R : Outport  VectorParamsAs1DForOutWhenUnconnected=off
  wires:
  Rcore/Lcore/1 -> Gain1/1
  Gain1/1 -> -Rm/Lm->(3,3)/2
  Rcore/1 -> Product1/1
  -Rm/Lm->(3,3)/1 -> R/1
  kRm->(3,2)/1 -> -Rm/Lm->(3,3)/1
  Product1/1 -> kRm->(3,2)/2
  k/1 -> Product1/2
  Gain/1 -> "-R2->(2,2) "/2
  Rin/1 -> "-R2->(2,2) "/1
  R2/1 -> Gain/1
  "-R2->(2,2) "/1 -> kRm->(3,2)/1

== system IEEE13bus_1subsystem/SM_13p/Regulator 1/Single Phase SVR_A2/Transformer with Taps/SSN OLTC xfo v2/conn_down_c ==
  b2 : PMIOPort  Side=Right
  b1 : PMIOPort  Port=2  Side=Left
  connections:
  b1/RConn1 -- b2/RConn1

== system IEEE13bus_1subsystem/SM_13p/Regulator 1/Single Phase SVR_A2/Transformer with Taps/SSN OLTC xfo v2/conn_down_d ==
  b2 : PMIOPort  Side=Right
  b1 : PMIOPort  Port=2  Side=Left
  connections:
  b1/RConn1 -- b2/RConn1

== system IEEE13bus_1subsystem/SM_13p/Regulator 1/Single Phase SVR_A2/Transformer with Taps/SSN OLTC xfo v2/conn_up_c ==
  b2 : PMIOPort  Side=Right
  b1 : PMIOPort  Port=2  Side=Left
  connections:
  b1/RConn1 -- b2/RConn1

== system IEEE13bus_1subsystem/SM_13p/Regulator 1/Single Phase SVR_A2/Transformer with Taps/SSN OLTC xfo v2/conn_up_d ==
  b2 : PMIOPort  Side=Right
  b1 : PMIOPort  Port=2  Side=Left
  connections:
  b1/RConn1 -- b2/RConn1

== system IEEE13bus_1subsystem/SM_13p/Regulator 1/Single Phase SVR_A2/Voltage Regulator Control/Tap Changer Control/Determine tap position ==
  NewTap : Inport
  Trigger : TriggerPort  VariantControl=Variant
  Memory : Memory  InitialCondition=InitialPosition  InheritSampleTime=on
  Saturation : Saturate  UpperLimit=MinMaxTap(2)  LowerLimit=MinMaxTap(1)
  Sum : Sum  Inputs=|++  SaturateOnIntegerOverflow=on
  TapNo : Outport  InitialOutput=InitialPosition  VectorParamsAs1DForOutWhenUnconnected=off
  wires:
  NewTap/1 -> Sum/1
  Sum/1 -> Saturation/1
  Memory/1 -> Sum/2
  Saturation/1 -> TapNo/1, Memory/1

== system IEEE13bus_1subsystem/SM_13p/Regulator 1/Single Phase SVR_A2/Voltage Regulator Control/Tap Changer Control/Edge Detector ==
  note: Edge or Slope Detector
  In : Inport
  Constant1 : Constant  Value=model
  Demux : Demux  Outputs=2
      settings: DisplayOption=none
  Logical Operator1 : Logic  Operator=OR
  Memory : Memory  InitialCondition=ic  LinearizeAsDelay=on
  Multiport Switch : MultiPortSwitch  InputSameDT=off
  NEGATIVE Edge : Subsystem  TreatAsAtomicUnit=on
  POSITIVE Edge : Subsystem  TreatAsAtomicUnit=on
  either edge : Constant  Value=[1 1]
  neg. edge : Constant  Value=[0 1]
  pos. edge : Constant  Value=[1 0]
  Out : Outport  VectorParamsAs1DForOutWhenUnconnected=off
  wires:
  either edge/1 -> Multiport Switch/4
  Demux/2 -> NEGATIVE Edge/Enable
  Demux/1 -> POSITIVE Edge/Enable
  Multiport Switch/1 -> Demux/1
  Constant1/1 -> Multiport Switch/1
  neg. edge/1 -> Multiport Switch/3
  pos. edge/1 -> Multiport Switch/2
  In/1 -> Memory/1, NEGATIVE Edge/1(IN), POSITIVE Edge/1(IN)
  Memory/1 -> NEGATIVE Edge/2(IN previous), POSITIVE Edge/2(IN previous)
  POSITIVE Edge/1(OUT) -> Logical Operator1/1
  NEGATIVE Edge/1(OUT) -> Logical Operator1/2
  Logical Operator1/1 -> Out/1

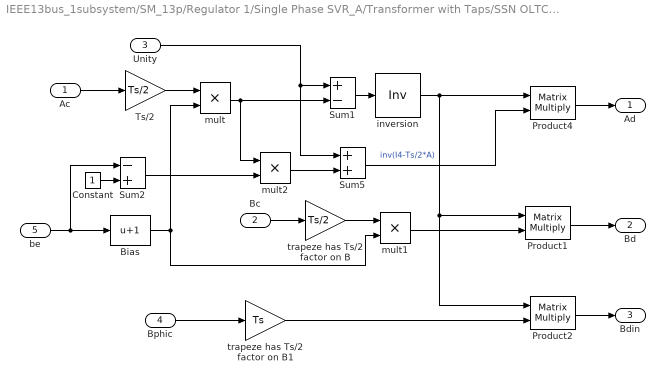
== system IEEE13bus_1subsystem/SM_13p/Regulator 1/Single Phase SVR_A/Transformer with Taps/SSN OLTC xfo v2/SSS-SM equations/Discretize ==
  Ac : Inport
  Bc : Inport  Port=2
  Unity : Inport  Port=3
  Bphic : Inport  Port=4
  be : Inport  Port=5
  Bias : Bias  Bias=1  SaturateOnIntegerOverflow=off
  Constant : Constant
  Product1 : Product  Multiplication=Matrix(*)  SaturateOnIntegerOverflow=on  OutDataTypeStr=Inherit: Same as first input
  Product2 : Product  Multiplication=Matrix(*)  SaturateOnIntegerOverflow=on  OutDataTypeStr=Inherit: Same as first input
  Product4 : Product  Multiplication=Matrix(*)  SaturateOnIntegerOverflow=on  OutDataTypeStr=Inherit: Same as first input
  Sum1 : Sum  Inputs=+-  SaturateOnIntegerOverflow=on
  Sum2 : Sum  Inputs=-+  SaturateOnIntegerOverflow=on
  Sum5 : Sum  SaturateOnIntegerOverflow=on
  Ts/2 : Gain  Gain=Ts/2  SaturateOnIntegerOverflow=on  OutDataTypeStr=Inherit: Same as input  ParamDataTypeStr=Inherit: Same as input
  inversion : Product  Inputs=/  Multiplication=Matrix(*)  RndMeth=Zero
  mult : Product
  mult1 : Product
  mult2 : Product
  trapeze has Ts/2 factor on B : Gain  Gain=Ts/2  SaturateOnIntegerOverflow=on  OutDataTypeStr=Inherit: Same as input  ParamDataTypeStr=Inherit: Same as input
  trapeze has Ts/2 factor on B1 : Gain  Gain=Ts  SaturateOnIntegerOverflow=on  OutDataTypeStr=Inherit: Same as input  ParamDataTypeStr=Inherit: Same as input
  Ad : Outport  VectorParamsAs1DForOutWhenUnconnected=off
  Bd : Outport  Port=2  VectorParamsAs1DForOutWhenUnconnected=off
  Bdin : Outport  Port=3  VectorParamsAs1DForOutWhenUnconnected=off
  wires:
  Sum2/1 -> mult2/2
  Constant/1 -> Sum2/2
  mult2/1 -> Sum5/2
  mult1/1 -> Product1/2
  trapeze has Ts/2 factor on B/1 -> mult1/1
  Bias/1 -> mult1/2, mult/2
  be/1 -> Sum2/1, Bias/1
  mult/1 -> mult2/1, Sum1/2
  Bphic/1 -> trapeze has Ts/2 factor on B1/1
  trapeze has Ts/2 factor on B1/1 -> Product2/2
  Product2/1 -> Bdin/1
  inversion/1 -> Product2/1, Product1/1, Product4/1  "inv(I4-Ts/2*A)"
  Bc/1 -> trapeze has Ts/2 factor on B/1
  Ts/2/1 -> mult/1
  Product4/1 -> Ad/1
  Unity/1 -> Sum5/1, Sum1/1
  Sum5/1 -> Product4/2
  Product1/1 -> Bd/1
  Ac/1 -> Ts/2/1
  Sum1/1 -> inversion/1

== system IEEE13bus_1subsystem/SM_13p/Regulator 1/Single Phase SVR_A/Voltage Regulator Control/Tap Changer Control/Edge Detector/NEGATIVE Edge ==
  IN : Inport
  IN previous : Inport  Port=2
  Enable : EnablePort  PropagateVarSize=During execution
  Relational Operator1 : RelationalOperator  Operator=>
  OUT : Outport  VectorParamsAs1DForOutWhenUnconnected=off
  wires:
  IN/1 -> Relational Operator1/2
  IN previous/1 -> Relational Operator1/1
  Relational Operator1/1 -> OUT/1

== system IEEE13bus_1subsystem/SM_13p/Regulator 1/Single Phase SVR_A/Voltage Regulator Control/Tap Changer Control/Edge Detector/POSITIVE Edge ==
  IN : Inport
  IN previous : Inport  Port=2
  Enable : EnablePort  PropagateVarSize=During execution
  Relational Operator1 : RelationalOperator  Operator=>
  OUT : Outport  VectorParamsAs1DForOutWhenUnconnected=off
  wires:
  IN/1 -> Relational Operator1/1
  IN previous/1 -> Relational Operator1/2
  Relational Operator1/1 -> OUT/1

== system IEEE13bus_1subsystem/SM_13p/Regulator 1/Single Phase SVR_A1/Transformer with Taps/SSN OLTC xfo v2/SSS-SM equations/Discretize ==
  Ac : Inport
  Bc : Inport  Port=2
  Unity : Inport  Port=3
  Bphic : Inport  Port=4
  be : Inport  Port=5
  Bias : Bias  Bias=1  SaturateOnIntegerOverflow=off
  Constant : Constant
  Product1 : Product  Multiplication=Matrix(*)  SaturateOnIntegerOverflow=on  OutDataTypeStr=Inherit: Same as first input
  Product2 : Product  Multiplication=Matrix(*)  SaturateOnIntegerOverflow=on  OutDataTypeStr=Inherit: Same as first input
  Product4 : Product  Multiplication=Matrix(*)  SaturateOnIntegerOverflow=on  OutDataTypeStr=Inherit: Same as first input
  Sum1 : Sum  Inputs=+-  SaturateOnIntegerOverflow=on
  Sum2 : Sum  Inputs=-+  SaturateOnIntegerOverflow=on
  Sum5 : Sum  SaturateOnIntegerOverflow=on
  Ts/2 : Gain  Gain=Ts/2  SaturateOnIntegerOverflow=on  OutDataTypeStr=Inherit: Same as input  ParamDataTypeStr=Inherit: Same as input
  inversion : Product  Inputs=/  Multiplication=Matrix(*)  RndMeth=Zero
  mult : Product
  mult1 : Product
  mult2 : Product
  trapeze has Ts/2 factor on B : Gain  Gain=Ts/2  SaturateOnIntegerOverflow=on  OutDataTypeStr=Inherit: Same as input  ParamDataTypeStr=Inherit: Same as input
  trapeze has Ts/2 factor on B1 : Gain  Gain=Ts  SaturateOnIntegerOverflow=on  OutDataTypeStr=Inherit: Same as input  ParamDataTypeStr=Inherit: Same as input
  Ad : Outport  VectorParamsAs1DForOutWhenUnconnected=off
  Bd : Outport  Port=2  VectorParamsAs1DForOutWhenUnconnected=off
  Bdin : Outport  Port=3  VectorParamsAs1DForOutWhenUnconnected=off
  wires:
  Sum1/1 -> inversion/1
  Ac/1 -> Ts/2/1
  Product1/1 -> Bd/1
  Sum5/1 -> Product4/2
  Unity/1 -> Sum1/1, Sum5/1
  Product4/1 -> Ad/1
  Ts/2/1 -> mult/1
  Bc/1 -> trapeze has Ts/2 factor on B/1
  inversion/1 -> Product4/1, Product1/1, Product2/1  "inv(I4-Ts/2*A)"
  Product2/1 -> Bdin/1
  trapeze has Ts/2 factor on B1/1 -> Product2/2
  Bphic/1 -> trapeze has Ts/2 factor on B1/1
  mult/1 -> Sum1/2, mult2/1
  be/1 -> Bias/1, Sum2/1
  Bias/1 -> mult/2, mult1/2
  trapeze has Ts/2 factor on B/1 -> mult1/1
  mult1/1 -> Product1/2
  mult2/1 -> Sum5/2
  Constant/1 -> Sum2/2
  Sum2/1 -> mult2/2

== system IEEE13bus_1subsystem/SM_13p/Regulator 1/Single Phase SVR_A1/Voltage Regulator Control/Tap Changer Control/Edge Detector/NEGATIVE Edge ==
  IN : Inport
  IN previous : Inport  Port=2
  Enable : EnablePort  PropagateVarSize=During execution
  Relational Operator1 : RelationalOperator  Operator=>
  OUT : Outport  VectorParamsAs1DForOutWhenUnconnected=off
  wires:
  Relational Operator1/1 -> OUT/1
  IN previous/1 -> Relational Operator1/1
  IN/1 -> Relational Operator1/2

== system IEEE13bus_1subsystem/SM_13p/Regulator 1/Single Phase SVR_A1/Voltage Regulator Control/Tap Changer Control/Edge Detector/POSITIVE Edge ==
  IN : Inport
  IN previous : Inport  Port=2
  Enable : EnablePort  PropagateVarSize=During execution
  Relational Operator1 : RelationalOperator  Operator=>
  OUT : Outport  VectorParamsAs1DForOutWhenUnconnected=off
  wires:
  Relational Operator1/1 -> OUT/1
  IN previous/1 -> Relational Operator1/2
  IN/1 -> Relational Operator1/1

== system IEEE13bus_1subsystem/SM_13p/Regulator 1/Single Phase SVR_A2/Transformer with Taps/SSN OLTC xfo v2/SSS-SM equations/Discretize ==
  Ac : Inport
  Bc : Inport  Port=2
  Unity : Inport  Port=3
  Bphic : Inport  Port=4
  be : Inport  Port=5
  Bias : Bias  Bias=1  SaturateOnIntegerOverflow=off
  Constant : Constant
  Product1 : Product  Multiplication=Matrix(*)  SaturateOnIntegerOverflow=on  OutDataTypeStr=Inherit: Same as first input
  Product2 : Product  Multiplication=Matrix(*)  SaturateOnIntegerOverflow=on  OutDataTypeStr=Inherit: Same as first input
  Product4 : Product  Multiplication=Matrix(*)  SaturateOnIntegerOverflow=on  OutDataTypeStr=Inherit: Same as first input
  Sum1 : Sum  Inputs=+-  SaturateOnIntegerOverflow=on
  Sum2 : Sum  Inputs=-+  SaturateOnIntegerOverflow=on
  Sum5 : Sum  SaturateOnIntegerOverflow=on
  Ts/2 : Gain  Gain=Ts/2  SaturateOnIntegerOverflow=on  OutDataTypeStr=Inherit: Same as input  ParamDataTypeStr=Inherit: Same as input
  inversion : Product  Inputs=/  Multiplication=Matrix(*)  RndMeth=Zero
  mult : Product
  mult1 : Product
  mult2 : Product
  trapeze has Ts/2 factor on B : Gain  Gain=Ts/2  SaturateOnIntegerOverflow=on  OutDataTypeStr=Inherit: Same as input  ParamDataTypeStr=Inherit: Same as input
  trapeze has Ts/2 factor on B1 : Gain  Gain=Ts  SaturateOnIntegerOverflow=on  OutDataTypeStr=Inherit: Same as input  ParamDataTypeStr=Inherit: Same as input
  Ad : Outport  VectorParamsAs1DForOutWhenUnconnected=off
  Bd : Outport  Port=2  VectorParamsAs1DForOutWhenUnconnected=off
  Bdin : Outport  Port=3  VectorParamsAs1DForOutWhenUnconnected=off
  wires:
  Sum2/1 -> mult2/2
  Constant/1 -> Sum2/2
  mult2/1 -> Sum5/2
  mult1/1 -> Product1/2
  trapeze has Ts/2 factor on B/1 -> mult1/1
  Bias/1 -> mult1/2, mult/2
  be/1 -> Sum2/1, Bias/1
  mult/1 -> mult2/1, Sum1/2
  Bphic/1 -> trapeze has Ts/2 factor on B1/1
  trapeze has Ts/2 factor on B1/1 -> Product2/2
  Product2/1 -> Bdin/1
  inversion/1 -> Product2/1, Product1/1, Product4/1  "inv(I4-Ts/2*A)"
  Bc/1 -> trapeze has Ts/2 factor on B/1
  Ts/2/1 -> mult/1
  Product4/1 -> Ad/1
  Unity/1 -> Sum5/1, Sum1/1
  Sum5/1 -> Product4/2
  Product1/1 -> Bd/1
  Ac/1 -> Ts/2/1
  Sum1/1 -> inversion/1

== system IEEE13bus_1subsystem/SM_13p/Regulator 1/Single Phase SVR_A2/Voltage Regulator Control/Tap Changer Control/Edge Detector/NEGATIVE Edge ==
  IN : Inport
  IN previous : Inport  Port=2
  Enable : EnablePort  PropagateVarSize=During execution
  Relational Operator1 : RelationalOperator  Operator=>
  OUT : Outport  VectorParamsAs1DForOutWhenUnconnected=off
  wires:
  IN/1 -> Relational Operator1/2
  IN previous/1 -> Relational Operator1/1
  Relational Operator1/1 -> OUT/1

== system IEEE13bus_1subsystem/SM_13p/Regulator 1/Single Phase SVR_A2/Voltage Regulator Control/Tap Changer Control/Edge Detector/POSITIVE Edge ==
  IN : Inport
  IN previous : Inport  Port=2
  Enable : EnablePort  PropagateVarSize=During execution
  Relational Operator1 : RelationalOperator  Operator=>
  OUT : Outport  VectorParamsAs1DForOutWhenUnconnected=off
  wires:
  IN/1 -> Relational Operator1/1
  IN previous/1 -> Relational Operator1/2
  Relational Operator1/1 -> OUT/1
